simulink model "Furnace"  (R2020a)
settings: Solver=ode15s  StartTime=0  StopTime=27000  FixedStep=0.1  MaxStep=20  MinStep=1e-13  RelTol=1e-08  AbsTol=1e-09
undefined symbols (not defined in the file): agnostic_lqe_params, cont_reg, disturbance_type, F_aI_pid, F_aII_pid, input_type, k, lqe_params, LQR_params, LQRAgnostic_params, MPC_type, MPCDiscrete_function_parameters, MPCDiscreteAgnostic_function_parameters, MPCDiscreteDiffIntegralAgnostic_function_parameters, original_LQR_params, output_type, reg, single_butter_ss
libraries: simulink x35, cstblocks x10, mpclib x3
(part 2 of 8)

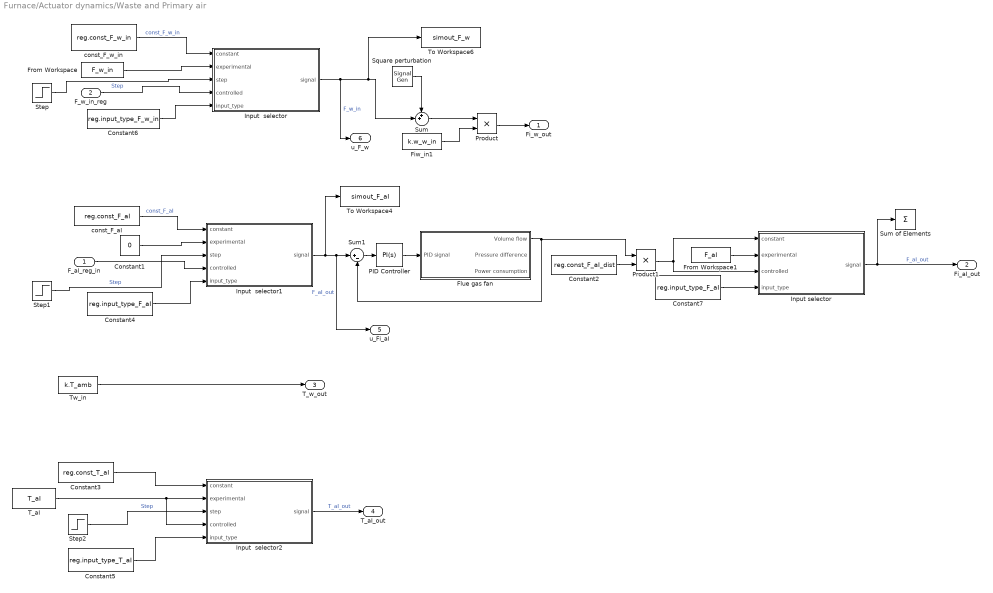
== system Furnace/Actuator dynamics/Waste and Primary air ==
  "F_aI_reg_in " : Inport
  F_w_in_reg : Inport  Port=2
  Constant1 : Constant  Value=0
  Constant2 : Constant  Value=reg.const_F_aI_dist
  Constant3 : Constant  Value=reg.const_T_aI
  Constant4 : Constant  Value=reg.input_type_F_aI
  Constant5 : Constant  Value=reg.input_type_T_aI
  Constant6 : Constant  Value=reg.input_type_F_w_in
  Constant7 : Constant  Value=reg.input_type_F_aI
  Fiw_in1 : Constant  Value=k.w_w_in
  Flue gas fan : Subsystem
  From Workspace : FromWorkspace  VariableName=F_w_in
  From Workspace1 : FromWorkspace  VariableName=F_aI
  Input  selector : MATLAB Function  TreatAsAtomicUnit=on
  Input  selector1 : MATLAB Function  TreatAsAtomicUnit=on
  Input  selector2 : MATLAB Function  TreatAsAtomicUnit=on
  Input selector : MATLAB Function  TreatAsAtomicUnit=on
  PID Controller : simulink/Continuous/PID Controller  Controller=PI  Form=Parallel  TimeDomain=Continuous-time  UseExternalTs=off  SampleTime=1  IntegratorMethod=Forward Euler  FilterMethod=Forward Euler  ControllerParametersSource=internal  P=reg.Kp_fan  I=reg.Ki_fan  D=0  UseFilter=on  N=100  TunerSelectOption=Transfer Function Based (PID Tuner App)  InitialConditionSource=internal  InitialConditionForIntegrator=reg.F_aI_fan_PID_int  InitialConditionForFilter=0  DifferentiatorICPrevScaledInput=0  ExternalReset=none  TrackingMode=off  Kt=1  LimitOutput=off  UpperSaturationLimit=inf  LowerSaturationLimit=-inf  LinearizeAsGain=on  AntiWindupMode=none  Kb=1  POutMin=[]  POutMax=[]  IOutMin=[]  IOutMax=[]  DOutMin=[]  DOutMax=[]  NOutMin=[]  NOutMax=[]  SumOutMin=[]  SumOutMax=[]  SaturationOutMin=[]  SaturationOutMax=[]  PParamMin=[]  PParamMax=[]  IParamMin=[]  IParamMax=[]  DParamMin=[]  DParamMax=[]  NParamMin=[]  NParamMax=[]  KbParamMin=[]  KbParamMax=[]  KtParamMin=[]  KtParamMax=[]  KbOutMin=[]  KbOutMax=[]  KtOutMin=[]  KtOutMax=[]  IntegratorOutMin=[]  IntegratorOutMax=[]  FilterOutMin=[]  FilterOutMax=[]  SumI1OutMin=[]  SumI1OutMax=[]  SumI2OutMin=[]  SumI2OutMax=[]  SumI3OutMin=[]  SumI3OutMax=[]  SumI4OutMin=[]  SumI4OutMax=[]  SumDOutMin=[]  SumDOutMax=[]  DifferentiatorOutMin=[]  DifferentiatorOutMax=[]  FilterDiffOutCoefMin=[]  FilterDiffOutCoefMax=[]  ReciprocalOutMin=[]  ReciprocalOutMax=[]  SumDenOutMin=[]  SumDenOutMax=[]  SumNumOutMin=[]  SumNumOutMax=[]  DivideOutMin=[]  DivideOutMax=[]  UdiffTsProdOutMin=[]  UdiffTsProdOutMax=[]  NTsProdOutMin=[]  NTsProdOutMax=[]  UintegralTsProdOutMin=[]  UintegralTsProdOutMax=[]  UngainTsProdOutMin=[]  UngainTsProdOutMax=[]  IntegratorContinuousStateAttributes=''  IntegratorStateMustResolveToSignalObject=off  IntegratorRTWStateStorageClass=Auto  FilterContinuousStateAttributes=''  FilterStateMustResolveToSignalObject=off  FilterRTWStateStorageClass=Auto  ParallelPVariant=InternalParameters  IdealPVariant=Disabled  IVariant=InternalParameters  DVariant=Disabled  IntegratorVariant=Continuous  SatVariant=Disabled  AWVariant=Passthrough  PCopyVariant=Disabled  TRVariant=Disabled  FdbkBlocksVariant=Forward  IdealPFdbkVariant=Disabled  SatFdbkVariant=Disabled  DerivativeFilterVariant=Disabled  NVariant=Disabled  NCopyVariant=Disabled_SignalSpec  FilterICVariant=Disabled  IntegratorICVariant=InternalICs  ExternalResetVariant=Disabled  TRSumVariant=Passthrough  SumFdbkVariant=Disabled  SumVariant=Sum_PI  TsampFilterVariant=InternalTs  TsampNgainVariant=Passthrough  TsampIntegralVariant=Passthrough
  Product : Product
  Product1 : Product
  Square perturbation : SignalGenerator  WaveForm=square  Amplitude=reg.F_w_pert_amp  Frequency=reg.F_w_pert_freq
  Step : Step  Time=reg.stepTime  Before=reg.const_F_w_in  After=reg.const_F_w_in_post_step  SampleTime=0
  Step1 : Step  Time=reg.stepTime  Before=reg.const_F_aI  After=reg.const_F_aI_post_step  SampleTime=0
  Step2 : Step  Time=reg.stepTime  Before=reg.const_T_aI  After=reg.const_T_aI_post_step  SampleTime=0
  Sum : Sum  Inputs=++|
  Sum of Elements : Sum  Inputs=+
  Sum1 : Sum  Inputs=|+-
  T_aI : FromWorkspace  VariableName=T_aI
  To Workspace4 : ToWorkspace  VariableName=simout_F_aI  SaveFormat=Timeseries  SampleTime=-1
  To Workspace6 : ToWorkspace  VariableName=simout_F_w  SaveFormat=Timeseries  SampleTime=-1
  Tw_in : Constant  Value=k.T_amb
  const_F_aI : Constant  Value=reg.const_F_aI
  const_F_w_in : Constant  Value=reg.const_F_w_in
  Fi_w_out : Outport  VectorParamsAs1DForOutWhenUnconnected=off
  Fi_aI_out : Outport  Port=2  VectorParamsAs1DForOutWhenUnconnected=off
  T_w_out : Outport  Port=3  VectorParamsAs1DForOutWhenUnconnected=off
  T_aI_out : Outport  Port=4  VectorParamsAs1DForOutWhenUnconnected=off
  u_Fi_aI : Outport  Port=5  VectorParamsAs1DForOutWhenUnconnected=off
  u_F_w : Outport  Port=6  VectorParamsAs1DForOutWhenUnconnected=off
  wires:
  Tw_in/1 -> T_w_out/1
  Fiw_in1/1 -> Product/2
  From Workspace/1 -> Input  selector/2(experimental)
  Product/1 -> Fi_w_out/1
  Input selector/1(signal) -> Fi_aI_out/1, Sum of Elements/1  "F_aI_out"
  From Workspace1/1 -> Input selector/2(experimental)
  Constant4/1 -> Input  selector1/5(input_type)
  Constant5/1 -> Input  selector2/5(input_type)
  T_aI/1 -> Input  selector2/4(controlled), Input  selector2/2(experimental)
  Constant3/1 -> Input  selector2/1(constant)
  Input  selector2/1(signal) -> T_aI_out/1  "T_aI_out"
  Constant6/1 -> Input  selector/5(input_type)
  F_w_in_reg/1 -> Input  selector/4(controlled)
  const_F_w_in/1 -> Input  selector/1(constant)  "const_F_w_in"
  Input  selector/1(signal) -> u_F_w/1, To Workspace6/1, Sum/2  "F_w_in"
  Sum/1 -> Product/1
  Square perturbation/1 -> Sum/1
  PID Controller/1 -> Flue gas fan/1(PID signal)
  Sum1/1 -> PID Controller/1
  const_F_aI/1 -> Input  selector1/1(constant)  "const_F_aI"
  "F_aI_reg_in "/1 -> Input  selector1/4(controlled)
  Constant1/1 -> Input  selector1/2(experimental)
  Constant2/1 -> Product1/2
  Product1/1 -> Input selector/1(constant), Input selector/3(controlled)
  Constant7/1 -> Input selector/4(input_type)
  Flue gas fan/1(Volume flow) -> Sum1/2, Product1/1
  Input  selector1/1(signal) -> To Workspace4/1, u_Fi_aI/1, Sum1/1  "F_aI_out"
  Step/1 -> Input  selector/3(step)  "Step"
  Step1/1 -> Input  selector1/3(step)  "Step"
  Step2/1 -> Input  selector2/3(step)  "Step"

== system Furnace/Controller/Butterworth_filter3 ==
  In : Inport
  Gain2 : Gain  Gain=single_butter_ss.B  Multiplication=Matrix(K*u)
  Gain3 : Gain  Gain=single_butter_ss.C  Multiplication=Matrix(K*u)
  Gain4 : Gain  Gain=single_butter_ss.A  Multiplication=Matrix(K*u)
  Integrator : Integrator
  Sum : Sum  Inputs=|++
  Filtered : Outport
  wires:
  Gain3/1 -> Filtered/1
  In/1 -> Gain2/1
  Gain2/1 -> Sum/1
  Integrator/1 -> Gain4/1, Gain3/1
  Gain4/1 -> Sum/2
  Sum/1 -> Integrator/1

== system Furnace/Controller/MPC_subsystem ==
  F_O2_in : Inport
  F_st_in : Inport  Port=2
  HHV_in : Inport  Port=3
  used_inputs : Inport  Port=4
  "\"Measured\" disturbances" : Inport  Port=5
  Constant1 : Constant  Value=lqe_params.u_star
  Constant11 : Constant  Value=lqe_params.y_star
  Constant2 : Constant  Value=lqe_params.u_star
  Constant3 : Constant  Value=lqe_params.v_star
  Demux1 : Demux
  LQG_controller : Subsystem
  MPC-ref : Constant  Value=[0;0]
  Mux2 : Mux  Inputs=3
  Revert to Summer ordering : Selector  InputPortWidth=4  IndexOptions=Index vector (dialog)  Indices=[1 3 4 2]  OutputSizes=1
  Scope{,1..4} (5 alike) : Scope
  Scope6 : Scope  Commented=on
  Selector : Selector  InputPortWidth=3  IndexOptions=Index vector (dialog)  Indices=[2 1 3]  OutputSizes=1
  Selector1 : Selector  InputPortWidth=3  IndexOptions=Index vector (dialog)  Indices=1:2  OutputSizes=1
  Selector5 : Selector  Commented=on  InputPortWidth=3  IndexOptions=Index vector (dialog)  Indices=1:2  OutputSizes=1
  Selector6 : Selector  InputPortWidth=5  IndexOptions=Index vector (dialog)  Indices=original_lqe_params.disturbance_measurement_indecies  OutputSizes=1
  Sine Wave : Sin  Commented=on  Amplitude=reg.include_noise * 1e-3  SampleTime=0
  Sum : Sum  Inputs=+-
  Sum1 : Sum  Inputs=|+-
  Sum2 : Sum  Inputs=|++
  Sum3 : Sum  Inputs=|+-
  Sum5 : Sum  Inputs=|+-
  Sum6 : Sum  Commented=on  Inputs=|-+
  Use internal ordering : Selector  InputPortWidth=4  IndexOptions=Index vector (dialog)  Indices=[1 4 2 3]  OutputSizes=1
  F_aII_MPC : Outport
  F_aI_MPC : Outport  Port=2
  v_grate_MPC : Outport  Port=3
  F_w_MPC : Outport  Port=4
  y_hat : Outport  Port=5
  wires:
  Demux1/1 -> F_aII_MPC/1
  Demux1/3 -> v_grate_MPC/1
  MPC-ref/1 -> LQG_controller/4(Controler_reference)
  Demux1/2 -> F_aI_MPC/1
  HHV_in/1 -> Mux2/3
  F_O2_in/1 -> Mux2/1
  F_st_in/1 -> Mux2/2
  Constant11/1 -> Sum1/2
  Demux1/4 -> F_w_MPC/1
  Sum2/1 -> Revert to Summer ordering/1
  Revert to Summer ordering/1 -> Demux1/1
  Selector/1 -> Sum1/1
  Selector1/1 -> Scope1/1  "MPC_y"
  Sum/1 -> Scope2/1
  Sum1/1 -> LQG_controller/1(noisy_y), Sum/2, Sum6/2, Selector1/1
  used_inputs/1 -> Use internal ordering/1
  Sum3/1 -> LQG_controller/3(u in)
  Constant2/1 -> Sum3/2
  Use internal ordering/1 -> Sum3/1
  Mux2/1 -> Selector/1
  Selector5/1 -> Scope6/1  "MPC_y"
  Sine Wave/1 -> Sum6/1
  Sum6/1 -> Selector5/1
  "\"Measured\" disturbances"/1 -> Selector6/1
  Constant3/1 -> Sum5/2
  Sum5/1 -> LQG_controller/2(v in), Scope4/1  "v in"
  Selector6/1 -> Sum5/1
  Constant1/1 -> Sum2/2
  LQG_controller/2(y_hat) -> y_hat/1, Scope3/1, Sum/1
  LQG_controller/1(u_mpc) -> Scope/1, Sum2/1

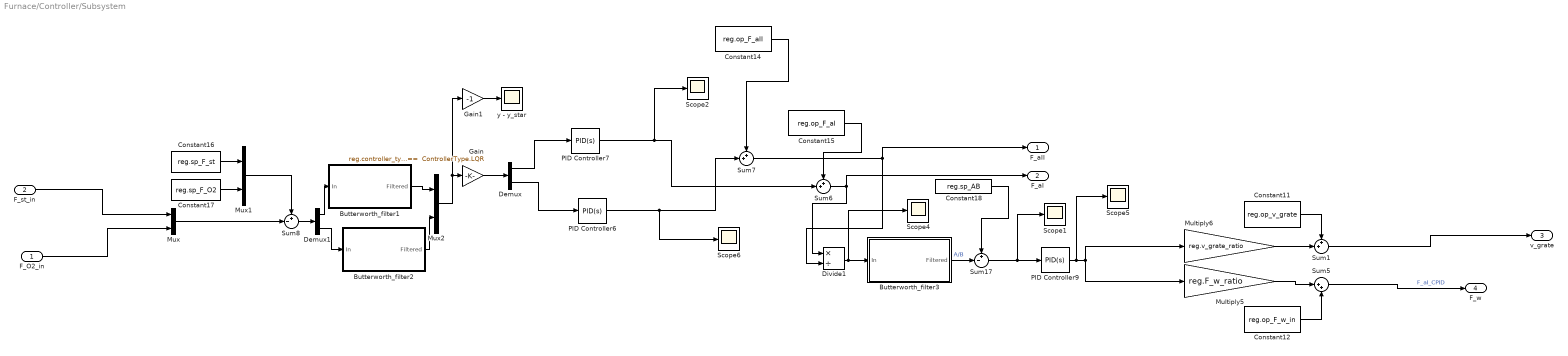
== system Furnace/Controller/Subsystem ==
  F_O2_in : Inport
  F_st_in : Inport  Port=2
  Butterworth_filter1 : Subsystem
  Butterworth_filter2 : Subsystem
  Butterworth_filter3 : Subsystem
  Constant11 : Constant  Value=reg.op_v_grate
  Constant12 : Constant  Value=reg.op_F_w_in
  Constant14 : Constant  Value=reg.op_F_aII
  Constant15 : Constant  Value=reg.op_F_aI
  Constant16 : Constant  Value=reg.sp_F_st
  Constant17 : Constant  Value=reg.sp_F_O2
  Constant18 : Constant  Value=reg.sp_AB
  Demux : Demux  Outputs=2
  Demux1 : Demux  Outputs=2
  Divide1 : Product  Inputs=*/
  Gain : Gain  Gain="reg.controller_type ==  ControllerType.LQR"
  Gain1 : Gain  Gain=-1
  Multiply5 : Gain  Gain=reg.F_w_ratio
  Multiply6 : Gain  Gain=reg.v_grate_ratio
  Mux : Mux  Inputs=2
  Mux1 : Mux  Inputs=2
  Mux2 : Mux  Inputs=2
  PID Controller6 : simulink/Continuous/PID Controller  Controller=PID  Form=Parallel  TimeDomain=Continuous-time  UseExternalTs=off  SampleTime=1  IntegratorMethod=Forward Euler  FilterMethod=Forward Euler  ControllerParametersSource=internal  P=F_aII_pid.Kp  I=F_aII_pid.Ki  D=F_aII_pid.Kd  UseFilter=on  N=100  TunerSelectOption=Transfer Function Based (PID Tuner App)  InitialConditionSource=internal  InitialConditionForIntegrator=0  InitialConditionForFilter=0  DifferentiatorICPrevScaledInput=0  ExternalReset=none  TrackingMode=off  Kt=1  LimitOutput=off  UpperSaturationLimit=inf  LowerSaturationLimit=1  LinearizeAsGain=on  AntiWindupMode=none  Kb=1  POutMin=[]  POutMax=[]  IOutMin=[]  IOutMax=[]  DOutMin=[]  DOutMax=[]  NOutMin=[]  NOutMax=[]  SumOutMin=[]  SumOutMax=[]  SaturationOutMin=[]  SaturationOutMax=[]  PParamMin=[]  PParamMax=[]  IParamMin=[]  IParamMax=[]  DParamMin=[]  DParamMax=[]  NParamMin=[]  NParamMax=[]  KbParamMin=[]  KbParamMax=[]  KtParamMin=[]  KtParamMax=[]  KbOutMin=[]  KbOutMax=[]  KtOutMin=[]  KtOutMax=[]  IntegratorOutMin=[]  IntegratorOutMax=[]  FilterOutMin=[]  FilterOutMax=[]  SumI1OutMin=[]  SumI1OutMax=[]  SumI2OutMin=[]  SumI2OutMax=[]  SumI3OutMin=[]  SumI3OutMax=[]  SumI4OutMin=[]  SumI4OutMax=[]  SumDOutMin=[]  SumDOutMax=[]  DifferentiatorOutMin=[]  DifferentiatorOutMax=[]  FilterDiffOutCoefMin=[]  FilterDiffOutCoefMax=[]  ReciprocalOutMin=[]  ReciprocalOutMax=[]  SumDenOutMin=[]  SumDenOutMax=[]  SumNumOutMin=[]  SumNumOutMax=[]  DivideOutMin=[]  DivideOutMax=[]  UdiffTsProdOutMin=[]  UdiffTsProdOutMax=[]  NTsProdOutMin=[]  NTsProdOutMax=[]  UintegralTsProdOutMin=[]  UintegralTsProdOutMax=[]  UngainTsProdOutMin=[]  UngainTsProdOutMax=[]  IntegratorContinuousStateAttributes='F_st'  IntegratorStateMustResolveToSignalObject=off  IntegratorRTWStateStorageClass=Auto  FilterContinuousStateAttributes=''  FilterStateMustResolveToSignalObject=off  FilterRTWStateStorageClass=Auto  ParallelPVariant=InternalParameters  IdealPVariant=Disabled  IVariant=InternalParameters  DVariant=InternalParameters  IntegratorVariant=Continuous  SatVariant=Disabled  AWVariant=Passthrough  PCopyVariant=Disabled  TRVariant=Disabled  FdbkBlocksVariant=Forward  IdealPFdbkVariant=Disabled  SatFdbkVariant=Disabled  DerivativeFilterVariant=ContFilter  NVariant=InternalParameters  NCopyVariant=Disabled  FilterICVariant=InternalICsFilter  IntegratorICVariant=InternalICs  ExternalResetVariant=Disabled  TRSumVariant=Passthrough  SumFdbkVariant=Disabled  SumVariant=Sum_PID  TsampFilterVariant=InternalTs  TsampNgainVariant=Passthrough  TsampIntegralVariant=Passthrough
  PID Controller7 : simulink/Continuous/PID Controller  Controller=PID  Form=Parallel  TimeDomain=Continuous-time  UseExternalTs=off  SampleTime=1  IntegratorMethod=Forward Euler  FilterMethod=Forward Euler  ControllerParametersSource=internal  P=F_aI_pid.Kp  I=F_aI_pid.Ki  D=F_aI_pid.Kd  UseFilter=on  N=100  TunerSelectOption=Transfer Function Based (PID Tuner App)  InitialConditionSource=internal  InitialConditionForIntegrator=0  InitialConditionForFilter=0  DifferentiatorICPrevScaledInput=0  ExternalReset=none  TrackingMode=off  Kt=1  LimitOutput=off  UpperSaturationLimit=inf  LowerSaturationLimit=1  LinearizeAsGain=on  AntiWindupMode=none  Kb=1  POutMin=[]  POutMax=[]  IOutMin=[]  IOutMax=[]  DOutMin=[]  DOutMax=[]  NOutMin=[]  NOutMax=[]  SumOutMin=[]  SumOutMax=[]  SaturationOutMin=[]  SaturationOutMax=[]  PParamMin=[]  PParamMax=[]  IParamMin=[]  IParamMax=[]  DParamMin=[]  DParamMax=[]  NParamMin=[]  NParamMax=[]  KbParamMin=[]  KbParamMax=[]  KtParamMin=[]  KtParamMax=[]  KbOutMin=[]  KbOutMax=[]  KtOutMin=[]  KtOutMax=[]  IntegratorOutMin=[]  IntegratorOutMax=[]  FilterOutMin=[]  FilterOutMax=[]  SumI1OutMin=[]  SumI1OutMax=[]  SumI2OutMin=[]  SumI2OutMax=[]  SumI3OutMin=[]  SumI3OutMax=[]  SumI4OutMin=[]  SumI4OutMax=[]  SumDOutMin=[]  SumDOutMax=[]  DifferentiatorOutMin=[]  DifferentiatorOutMax=[]  FilterDiffOutCoefMin=[]  FilterDiffOutCoefMax=[]  ReciprocalOutMin=[]  ReciprocalOutMax=[]  SumDenOutMin=[]  SumDenOutMax=[]  SumNumOutMin=[]  SumNumOutMax=[]  DivideOutMin=[]  DivideOutMax=[]  UdiffTsProdOutMin=[]  UdiffTsProdOutMax=[]  NTsProdOutMin=[]  NTsProdOutMax=[]  UintegralTsProdOutMin=[]  UintegralTsProdOutMax=[]  UngainTsProdOutMin=[]  UngainTsProdOutMax=[]  IntegratorContinuousStateAttributes='F_st'  IntegratorStateMustResolveToSignalObject=off  IntegratorRTWStateStorageClass=Auto  FilterContinuousStateAttributes=''  FilterStateMustResolveToSignalObject=off  FilterRTWStateStorageClass=Auto  ParallelPVariant=InternalParameters  IdealPVariant=Disabled  IVariant=InternalParameters  DVariant=InternalParameters  IntegratorVariant=Continuous  SatVariant=Disabled  AWVariant=Passthrough  PCopyVariant=Disabled  TRVariant=Disabled  FdbkBlocksVariant=Forward  IdealPFdbkVariant=Disabled  SatFdbkVariant=Disabled  DerivativeFilterVariant=ContFilter  NVariant=InternalParameters  NCopyVariant=Disabled  FilterICVariant=InternalICsFilter  IntegratorICVariant=InternalICs  ExternalResetVariant=Disabled  TRSumVariant=Passthrough  SumFdbkVariant=Disabled  SumVariant=Sum_PID  TsampFilterVariant=InternalTs  TsampNgainVariant=Passthrough  TsampIntegralVariant=Passthrough
  PID Controller9 : simulink/Continuous/PID Controller  Controller=PID  Form=Parallel  TimeDomain=Continuous-time  UseExternalTs=off  SampleTime=1  IntegratorMethod=Forward Euler  FilterMethod=Forward Euler  ControllerParametersSource=internal  P=F_aII_pid.Kp  I=F_aII_pid.Ki  D=F_aII_pid.Kd  UseFilter=on  N=100  TunerSelectOption=Transfer Function Based (PID Tuner App)  InitialConditionSource=internal  InitialConditionForIntegrator=0  InitialConditionForFilter=0  DifferentiatorICPrevScaledInput=0  ExternalReset=none  TrackingMode=off  Kt=1  LimitOutput=off  UpperSaturationLimit=inf  LowerSaturationLimit=1  LinearizeAsGain=on  AntiWindupMode=none  Kb=1  POutMin=[]  POutMax=[]  IOutMin=[]  IOutMax=[]  DOutMin=[]  DOutMax=[]  NOutMin=[]  NOutMax=[]  SumOutMin=[]  SumOutMax=[]  SaturationOutMin=[]  SaturationOutMax=[]  PParamMin=[]  PParamMax=[]  IParamMin=[]  IParamMax=[]  DParamMin=[]  DParamMax=[]  NParamMin=[]  NParamMax=[]  KbParamMin=[]  KbParamMax=[]  KtParamMin=[]  KtParamMax=[]  KbOutMin=[]  KbOutMax=[]  KtOutMin=[]  KtOutMax=[]  IntegratorOutMin=[]  IntegratorOutMax=[]  FilterOutMin=[]  FilterOutMax=[]  SumI1OutMin=[]  SumI1OutMax=[]  SumI2OutMin=[]  SumI2OutMax=[]  SumI3OutMin=[]  SumI3OutMax=[]  SumI4OutMin=[]  SumI4OutMax=[]  SumDOutMin=[]  SumDOutMax=[]  DifferentiatorOutMin=[]  DifferentiatorOutMax=[]  FilterDiffOutCoefMin=[]  FilterDiffOutCoefMax=[]  ReciprocalOutMin=[]  ReciprocalOutMax=[]  SumDenOutMin=[]  SumDenOutMax=[]  SumNumOutMin=[]  SumNumOutMax=[]  DivideOutMin=[]  DivideOutMax=[]  UdiffTsProdOutMin=[]  UdiffTsProdOutMax=[]  NTsProdOutMin=[]  NTsProdOutMax=[]  UintegralTsProdOutMin=[]  UintegralTsProdOutMax=[]  UngainTsProdOutMin=[]  UngainTsProdOutMax=[]  IntegratorContinuousStateAttributes='F_st'  IntegratorStateMustResolveToSignalObject=off  IntegratorRTWStateStorageClass=Auto  FilterContinuousStateAttributes=''  FilterStateMustResolveToSignalObject=off  FilterRTWStateStorageClass=Auto  ParallelPVariant=InternalParameters  IdealPVariant=Disabled  IVariant=InternalParameters  DVariant=InternalParameters  IntegratorVariant=Continuous  SatVariant=Disabled  AWVariant=Passthrough  PCopyVariant=Disabled  TRVariant=Disabled  FdbkBlocksVariant=Forward  IdealPFdbkVariant=Disabled  SatFdbkVariant=Disabled  DerivativeFilterVariant=ContFilter  NVariant=InternalParameters  NCopyVariant=Disabled  FilterICVariant=InternalICsFilter  IntegratorICVariant=InternalICs  ExternalResetVariant=Disabled  TRSumVariant=Passthrough  SumFdbkVariant=Disabled  SumVariant=Sum_PID  TsampFilterVariant=InternalTs  TsampNgainVariant=Passthrough  TsampIntegralVariant=Passthrough
  Scope{1..2,4..6} (5 alike) : Scope
  Sum1 : Sum  Inputs=++|
  Sum17 : Sum  Inputs=+-|
  Sum5 : Sum  Inputs=|++
  Sum6 : Sum  Inputs=++|
  Sum7 : Sum  Inputs=++|
  Sum8 : Sum  Inputs=+-|
  y - y_star : Scope
  F_aII : Outport
  F_aI : Outport  Port=2
  v_grate : Outport  Port=3
  F_w : Outport  Port=4
  wires:
  Gain/1 -> Demux/1
  Constant14/1 -> Sum7/1
  Demux1/2 -> Butterworth_filter2/1(In)
  PID Controller6/1 -> Scope6/1, Sum7/2
  PID Controller7/1 -> Scope2/1, Sum6/2
  Sum17/1 -> Scope1/1, PID Controller9/1
  Constant11/1 -> Sum1/1
  Constant18/1 -> Sum17/1
  Demux/2 -> PID Controller6/1
  Mux/1 -> Sum8/2
  Constant16/1 -> Mux1/1
  Multiply6/1 -> Sum1/2
  Constant15/1 -> Sum6/1
  Sum8/1 -> Demux1/1
  Sum6/1 -> F_aI/1, Divide1/1
  Constant17/1 -> Mux1/2
  Demux/1 -> PID Controller7/1
  Multiply5/1 -> Sum5/1
  Butterworth_filter3/1(Filtered) -> Sum17/2  "A/B"
  F_O2_in/1 -> Mux/2
  Sum1/1 -> v_grate/1
  Mux1/1 -> Sum8/1
  F_st_in/1 -> Mux/1
  PID Controller9/1 -> Scope5/1, Multiply5/1, Multiply6/1
  Sum7/1 -> F_aII/1, Divide1/2
  Sum5/1 -> F_w/1  "F_aI_CPID"
  Mux2/1 -> Gain1/1, Gain/1
  Butterworth_filter1/1(Filtered) -> Mux2/1
  Divide1/1 -> Butterworth_filter3/1(In), Scope4/1
  Demux1/1 -> Butterworth_filter1/1(In)
  Constant12/1 -> Sum5/2
  Butterworth_filter2/1(Filtered) -> Mux2/2
  Gain1/1 -> y - y_star/1

== system Furnace/Deprecated, slow loop/Actuator dynamics ==
  F_aII_reg_in : Inport
  F_w_in_reg : Inport  Port=2
  "F_aI_reg_in " : Inport  Port=3
  v_grate_reg_in : Inport  Port=4
  uncontrolled_variables : Inport  Port=5
  Bus Selector : BusSelector  OutputSignals=Q_grate,Tw,T_aI,T_aII
  Grate speed : Subsystem
  Secondary air : Subsystem
      mask Display: image('airflow.jpeg');
  Waste and Primary air : Subsystem
      mask Display: image('waste_in.jpg');
  v_grate : Outport
  Q_grate_out : Outport  Port=2
  Fi_w : Outport  Port=3
  Fi_aI : Outport  Port=4
  T_w : Outport  Port=5
  T_aI : Outport  Port=6
  F_aII_out : Outport  Port=7
  T_aII_out : Outport  Port=8
  wires:
  Grate speed/1(v_grate_out) -> v_grate/1  "v_grate"
  F_w_in_reg/1 -> Waste and Primary air/2(F_w_in_reg)
  Secondary air/1(F_aII_out) -> F_aII_out/1
  v_grate_reg_in/1 -> Grate speed/1(v_grate_reg_in)
  Waste and Primary air/1(Fi_w_out) -> Fi_w/1  "Fi_w"
  "F_aI_reg_in "/1 -> Waste and Primary air/1("F_aI_reg_in ")
  Waste and Primary air/2(Fi_aI_out) -> Fi_aI/1  "Fi_aI"
  F_aII_reg_in/1 -> Secondary air/1(F_aII_reg_in)
  uncontrolled_variables/1 -> Bus Selector/1
  Bus Selector/1 -> Q_grate_out/1  "<Q_grate>"
  Bus Selector/2 -> T_w/1  "<Tw>"
  Bus Selector/3 -> T_aI/1  "<T_aI>"
  Bus Selector/4 -> T_aII_out/1  "<T_aII>"

== system Furnace/Deprecated, slow loop/Constant disturbances ==
  Constant2 : Constant  Value=reg.const_T_aII
  Constant3 : Constant  Value=reg.const_T_aI
  Tw_in : Constant  Value=k.T_amb
  const_Q_grate : Constant  Value=reg.const_Q_grate
  Q_grate : Outport
  T_w : Outport  Port=2
  T_aI : Outport  Port=3
  T_aII : Outport  Port=4
  wires:
  Constant2/1 -> T_aII/1  "T_aII"
  const_Q_grate/1 -> Q_grate/1  "Q_grate"
  Tw_in/1 -> T_w/1  "Tw"
  Constant3/1 -> T_aI/1  "T_aI"

== system Furnace/Deprecated, slow loop/Constant inputs ==
  F_aII distribution : Gain  Gain=reg.const_F_aI_dist
  const_F_aI : Constant  Value=reg.const_F_aI
  const_F_aII : Constant  Value=reg.const_F_aII
  const_F_w_in : Constant  Value=reg.const_F_w_in
  const_v_grate : Constant  Value=reg.const_v_grate
  F_aII : Outport
  Fw : Outport  Port=2
  F_aI : Outport  Port=3
  v_grate : Outport  Port=4
  wires:
  const_v_grate/1 -> v_grate/1  "v_grate"
  const_F_aII/1 -> F_aII/1  "F_aII"
  const_F_aI/1 -> F_aII distribution/1  "F_aI"
  const_F_w_in/1 -> Fw/1  "F_w"
  F_aII distribution/1 -> F_aI/1  "F_aI"

== system Furnace/Deprecated, slow loop/Contineous Summer student feedback (Not finished) ==
  Fi_fg_in : Inport
  F_st_in : Inport  Port=2
  HHV_in : Inport  Port=3
  Controller : Subsystem
  Grate speed : Subsystem
  Secondary air : Subsystem
      mask Display: image('airflow.jpeg');
  Terminator{1..4} (4 alike) : Terminator
  Waste and Primary air : Subsystem
      mask Display: image('waste_in.jpg');
  F_aII_out : Outport
  Fi_w : Outport  Port=2
  Fi_aI : Outport  Port=3
  v_grate : Outport  Port=4
  wires:
  Controller/4(Fi_w_out) -> Waste and Primary air/2(F_w_in_reg)
  Controller/3(v_grate_out) -> Grate speed/1(v_grate_reg_in)
  Secondary air/1(F_aII_out) -> F_aII_out/1
  F_st_in/1 -> Controller/2(F_st_in)
  Fi_fg_in/1 -> Controller/1(Fi_fg_in)
  HHV_in/1 -> Controller/3(HHV_in)
  Grate speed/1(v_grate_out) -> v_grate/1  "v_grate"
  Controller/2(Fi_aI_out) -> Waste and Primary air/1("F_aI_reg_in ")
  Waste and Primary air/2(Fi_aI_out) -> Fi_aI/1  "Fi_aI"
  Controller/1(F_aII_out) -> Secondary air/1(F_aII_reg_in)
  Waste and Primary air/1(Fi_w_out) -> Fi_w/1  "Fi_w"
  Waste and Primary air/3(Fi_aI_out1) -> Terminator2/1
  Waste and Primary air/4(Fi_aI_out2) -> Terminator1/1
  Secondary air/2(F_aII_out1) -> Terminator3/1
  Grate speed/2(Q_grate_out) -> Terminator4/1

== system Furnace/Deprecated, slow loop/Controller ==
  F_st_in : Inport
  Fi_fg_in : Inport  Port=2
  HHV_in : Inport  Port=3
  Summer Controller (Cleaned) : Subsystem
  "Summer Controller (Old) " : Subsystem  Commented=on
  F_aII_out : Outport
  Fi_w_out : Outport  Port=2
  Full_Fi_aI_out : Outport  Port=3
  v_grate_out : Outport  Port=4
  wires:
  F_st_in/1 -> Summer Controller (Cleaned)/1(F_st_in)
  Fi_fg_in/1 -> Summer Controller (Cleaned)/2(Fi_O2_in)
  HHV_in/1 -> Summer Controller (Cleaned)/3(HHV_in)
  Summer Controller (Cleaned)/1(F_aII_out) -> F_aII_out/1
  Summer Controller (Cleaned)/3(Fi_aI_out) -> Full_Fi_aI_out/1
  Summer Controller (Cleaned)/2(Fi_w_out) -> Fi_w_out/1
  Summer Controller (Cleaned)/4(v_grate_out) -> v_grate_out/1

== system Furnace/Deprecated, slow loop/Experimental disturbances ==
  Constant  T_amb : Constant  Value=k.T_amb
  From Workspace2 : FromWorkspace  VariableName=Q_grate
  T_aII : FromWorkspace  VariableName=T_aII
  T_aI_w : FromWorkspace  VariableName=T_aI
  Q_grate1 : Outport
  T_w : Outport  Port=2
  T_aI1 : Outport  Port=3
  T_aII2 : Outport  Port=4
  wires:
  T_aII/1 -> T_aII2/1  "T_aII"
  From Workspace2/1 -> Q_grate1/1  "Q_grate"
  T_aI_w/1 -> T_aI1/1  "T_aI"
  Constant  T_amb/1 -> T_w/1  "Tw"

== system Furnace/Deprecated, slow loop/Experimental inputs ==
  Constant2 : Constant  Value=reg.const_F_aI_dist
  From Workspace : FromWorkspace  VariableName=F_w_in
  From Workspace1 : FromWorkspace  VariableName=F_aII
  From Workspace3 : FromWorkspace  VariableName=F_aI
  v_grate1 : Constant  Value=k.v_grate
  F_aII : Outport
  Fw : Outport  Port=2
  F_aI : Outport  Port=3
  v_grate : Outport  Port=4
  wires:
  From Workspace1/1 -> F_aII/1  "F_aII"
  From Workspace3/1 -> F_aI/1  "F_aI"
  v_grate1/1 -> v_grate/1  "v_grate"
  From Workspace/1 -> Fw/1  "F_w"

== system Furnace/Deprecated, slow loop/Furnace ==
  v_grate_in : Inport
  Q_grate_in : Inport  Port=2
  Fi_w_in : Inport  Port=3
  Fi_aI_in : Inport  Port=4
  T_w_in : Inport  Port=5
  T_aI_in : Inport  Port=6
  F_aII_in : Inport  Port=7
  T_aII_in : Inport  Port=8
  Ashes : Subsystem
      mask Display: image('ash.jpg');
  "Auxiliary \"burners\"" : Subsystem
      mask Display: image('burnerim.jpg');
  Boiler : Subsystem
      mask Display: image('Boiler.jpg');
  Bus Selector : BusSelector  OutputSignals=F_w_ash
  Calorific Value : Subsystem
  Cold water from district heating : Subsystem
      mask Display: image('fromdh.jpg');
  Condenser : Subsystem
      mask Display: image('Condenser.jpg');
  Flue-gas fan : Subsystem  Commented=on
      mask Display: image('Fan.jpg');
  Flue-gas stack : Subsystem  Commented=on
      mask Display: image('Stack.jpg');
  Free board : Subsystem
      mask Display: image('fbim.jpg');
  Gas cleaning systems : Subsystem  Commented=on
      mask Display: image('Cleaning.jpg');
  Grate : Subsystem
      settings: MinAlgLoopOccurrences=on
      mask Display: image('grateim.jpg');
  Hot water to district heating : Subsystem
      mask Display: image('todh.jpg');
  Scope : Scope
  Scope1 : Scope
  Scope2 : Scope
  Turbine : Subsystem
      mask Display: image('Turbine.jpg');
  F_st_out : Outport  VectorParamsAs1DForOutWhenUnconnected=off
  F_fg_out : Outport  Port=2  VectorParamsAs1DForOutWhenUnconnected=off
  HHV_out : Outport  Port=3  VectorParamsAs1DForOutWhenUnconnected=off
  wires:
  Boiler/3(p_drum) -> Turbine/3(p_drum)
  Free board/1(T_fg_out) -> Calorific Value/1(T_fg), Scope/1, Boiler/2(T_fg), Grate/1(T_rad), "Auxiliary \"burners\""/1(In1)  "T_rad"
  Turbine/1(F_turb) -> Condenser/2(F_turb)
  Grate/1(Fi_fg_from_grate) -> Ashes/1(In1), Free board/1(Fi_in)
  Q_grate_in/1 -> Grate/4(Q_grate)
  Condenser/1(T_district) -> Hot water to district heating/1(In1)
  Cold water from district heating/1(Out1) -> Condenser/1(F_district)
  Grate/2(T_w_grate) -> Ashes/2(In2), Free board/2(T_in)
  "Auxiliary \"burners\""/1(Out1) -> Scope1/1, Grate/2(Q_burners)  "Q_burners"
  Grate/4(Q_rad_fg) -> Free board/3(Q_rad)
  Free board/2(Fi_fg_to_boiler) -> F_fg_out/1, Calorific Value/2(Fi_fg), Boiler/3(F_fg)
  Flue-gas fan/1(Out1) -> Flue-gas stack/1(T_fg)
  Boiler/4(T_fg_out) -> Gas cleaning systems/1(T_fg)
  Boiler/2(F_SH) -> F_st_out/1, Turbine/2(F_SH)  "F_steam"
  Flue-gas fan/2(Out2) -> Flue-gas stack/2(Fi_fg)
  Grate/5(OutBus) -> Bus Selector/1, Ashes/3(InBus)
  Condenser/2(T_w_out) -> Boiler/1(T_fromHE)
  Gas cleaning systems/2(Fi_fg_clean) -> Flue-gas fan/2(Fi_fg)
  Boiler/1(T_SH) -> Turbine/1(T_SH)
  Free board/3(F_flyash_tot) -> Boiler/4(F_flyash)
  Grate/3(F_flyash) -> Free board/4(F_flyash_cell)
  Gas cleaning systems/1(T_fg_clean) -> Flue-gas fan/1(T_fg)
  v_grate_in/1 -> Grate/3(v_grate_in)
  Boiler/5(Fi_fg_out) -> Gas cleaning systems/2(F_fg)
  Condenser/3(F_cond) -> Boiler/5(F_ECO)
  Boiler/6(F_flyash_out) -> Gas cleaning systems/3(F_flyash)
  Cold water from district heating/2(Out2) -> Condenser/3(T_return)
  Calorific Value/1(HHV) -> HHV_out/1  "HHV"
  Fi_w_in/1 -> Grate/5(Fi_w_in)
  Fi_aI_in/1 -> Grate/6(F_aI_in)
  T_w_in/1 -> Grate/7(T_w_in)
  T_aI_in/1 -> Grate/8(T_aI_in)
  F_aII_in/1 -> Free board/5(F_aII_in)
  T_aII_in/1 -> Free board/6(T_aII_in)
  Bus Selector/1 -> Scope2/1  "<F_w_ash>"

== system Furnace/Plant2/Ashes ==
  In1 : Inport
  In2 : Inport  Port=2
  In Bus Element : Inport  Port=3  PortName=InBus  Element=M_w_grate
  In Bus Element1 : Inport  Port=3  PortName=InBus  Element=M_char
  In Bus Element2 : Inport  Port=3  PortName=InBus  Element=F_w_ash
  In Bus Element3 : Inport  Port=3  PortName=InBus  Element=F_char_ash
  Flow of char ash : Display
  Flow of waste ash : Display
  Mass of char in grate : Display
  Scope1 : Scope
  Sum of Elements : Sum  Inputs=+  CollapseMode=Specified dimension
  Temperatures in grate : Display
  Waste in grate (mass) : Display
  wires:
  In Bus Element2/1 -> Flow of waste ash/1
  In Bus Element/1 -> Waste in grate (mass)/1
  In Bus Element1/1 -> Mass of char in grate/1
  In Bus Element3/1 -> Flow of char ash/1
  In1/1 -> Sum of Elements/1
  In2/1 -> Temperatures in grate/1
  Sum of Elements/1 -> Scope1/1

== system Furnace/Plant2/Auxiliary "burners" ==
  In1 : Inport
  Constant : Constant  Value=0
  Constant1 : Constant  Value=850+k.T_amb
  Minus : Sum  Inputs=+-
  "Q " : Constant  Value=3.5e6
  Switch : Switch  Criteria=u2 > Threshold
  Out1 : Outport  VectorParamsAs1DForOutWhenUnconnected=off
  wires:
  Switch/1 -> Out1/1
  Constant/1 -> Switch/3
  "Q "/1 -> Switch/1
  Minus/1 -> Switch/2
  Constant1/1 -> Minus/1
  In1/1 -> Minus/2

== system Furnace/Plant2/Boiler ==
  T_fromHE : Inport
  T_fg : Inport  Port=2
  F_fg : Inport  Port=3
  F_flyash : Inport  Port=4
  F_ECO : Inport  Port=5
  Constant : Constant  Value=0
  Constant1 : Constant  Value=k.p_drum
  Constant2 : Constant  Value=k.p_drum
  Drum : Subsystem
      mask Display: image('Drum.jpg');
  Economizer : Subsystem
  Evaporator : Subsystem
  Gain : Gain  Gain=1e-5
  Goto : Goto  Commented=on  GotoTag=T_drum  TagVisibility=global
  MATLAB Function : MATLAB Function  TreatAsAtomicUnit=on
  PID Controller : simulink/Continuous/PID Controller  Controller=PID  Form=Parallel  TimeDomain=Continuous-time  UseExternalTs=off  SampleTime=-1  IntegratorMethod=Forward Euler  FilterMethod=Forward Euler  ControllerParametersSource=internal  P=10  I=0  D=0  UseFilter=on  N=100  TunerSelectOption=Transfer Function Based (PID Tuner App)  InitialConditionSource=internal  InitialConditionForIntegrator=0  InitialConditionForFilter=0  DifferentiatorICPrevScaledInput=0  ExternalReset=none  TrackingMode=off  Kt=1  LimitOutput=on  UpperSaturationLimit=50  LowerSaturationLimit=0  LinearizeAsGain=on  AntiWindupMode=none  Kb=1  POutMin=[]  POutMax=[]  IOutMin=[]  IOutMax=[]  DOutMin=[]  DOutMax=[]  NOutMin=[]  NOutMax=[]  SumOutMin=[]  SumOutMax=[]  SaturationOutMin=[]  SaturationOutMax=[]  PParamMin=[]  PParamMax=[]  IParamMin=[]  IParamMax=[]  DParamMin=[]  DParamMax=[]  NParamMin=[]  NParamMax=[]  KbParamMin=[]  KbParamMax=[]  KtParamMin=[]  KtParamMax=[]  KbOutMin=[]  KbOutMax=[]  KtOutMin=[]  KtOutMax=[]  IntegratorOutMin=[]  IntegratorOutMax=[]  FilterOutMin=[]  FilterOutMax=[]  SumI1OutMin=[]  SumI1OutMax=[]  SumI2OutMin=[]  SumI2OutMax=[]  SumI3OutMin=[]  SumI3OutMax=[]  SumI4OutMin=[]  SumI4OutMax=[]  SumDOutMin=[]  SumDOutMax=[]  DifferentiatorOutMin=[]  DifferentiatorOutMax=[]  FilterDiffOutCoefMin=[]  FilterDiffOutCoefMax=[]  ReciprocalOutMin=[]  ReciprocalOutMax=[]  SumDenOutMin=[]  SumDenOutMax=[]  SumNumOutMin=[]  SumNumOutMax=[]  DivideOutMin=[]  DivideOutMax=[]  UdiffTsProdOutMin=[]  UdiffTsProdOutMax=[]  NTsProdOutMin=[]  NTsProdOutMax=[]  UintegralTsProdOutMin=[]  UintegralTsProdOutMax=[]  UngainTsProdOutMin=[]  UngainTsProdOutMax=[]  IntegratorContinuousStateAttributes=''  IntegratorStateMustResolveToSignalObject=off  IntegratorRTWStateStorageClass=Auto  FilterContinuousStateAttributes=''  FilterStateMustResolveToSignalObject=off  FilterRTWStateStorageClass=Auto  ParallelPVariant=InternalParameters  IdealPVariant=Disabled  IVariant=InternalParameters  DVariant=InternalParameters  IntegratorVariant=Continuous  SatVariant=Enabled  AWVariant=Passthrough  PCopyVariant=Disabled  TRVariant=Disabled  FdbkBlocksVariant=Forward  IdealPFdbkVariant=Disabled  SatFdbkVariant=Disabled  DerivativeFilterVariant=ContFilter  NVariant=InternalParameters  NCopyVariant=Disabled  FilterICVariant=InternalICsFilter  IntegratorICVariant=InternalICs  ExternalResetVariant=Disabled  TRSumVariant=Passthrough  SumFdbkVariant=Disabled  SumVariant=Sum_PID  TsampFilterVariant=InternalTs  TsampNgainVariant=Passthrough  TsampIntegralVariant=Passthrough
  PID null saturator : Switch
  Scope : Scope
  Scope1 : Scope
  Scope2 : Scope
  Sum1 : Sum  Inputs=+-|
  Super heater : Subsystem
  x_vap : Scope
  T_SH : Outport  VectorParamsAs1DForOutWhenUnconnected=off
  F_SH : Outport  Port=2  PortDimensions=1  VectorParamsAs1DForOutWhenUnconnected=off
  p_drum : Outport  Port=3  VectorParamsAs1DForOutWhenUnconnected=off
  T_fg_out : Outport  Port=4  VectorParamsAs1DForOutWhenUnconnected=off
  Fi_fg_out : Outport  Port=5  VectorParamsAs1DForOutWhenUnconnected=off
  F_flyash_out : Outport  Port=6  VectorParamsAs1DForOutWhenUnconnected=off
  wires:
  Evaporator/3(Fi_fg_out) -> Super heater/4(Fi_fg)
  Super heater/4(Fi_fg_out) -> Economizer/3(Fi_fg)
  Super heater/3(T_fg_out) -> Economizer/2(T_fg)
  Evaporator/2(T_fg_out) -> Super heater/3(T_fg)
  Economizer/3(Fi_fg_out) -> Fi_fg_out/1
  F_fg/1 -> Evaporator/3(Fi_fg)
  T_fg/1 -> Evaporator/2(T_fg)
  Super heater/2(T_steam) -> T_SH/1
  Economizer/2(T_fg_out) -> T_fg_out/1
  Drum/3(p_drum) -> MATLAB Function/1(p_drum), Sum1/1, p_drum/1
  T_fromHE/1 -> Economizer/1(T_fromHE)
  Super heater/5(F_SH) -> F_SH/1
  Drum/2(x_vap) -> x_vap/1
  PID Controller/1 -> Drum/3(F_vap), Scope/1, Super heater/1(F_steam)
  Constant1/1 -> Sum1/2
  Constant/1 -> PID null saturator/3
  Sum1/1 -> Gain/1
  [Q_cleaning] -> Drum/5(Q_cleaning)
  F_flyash/1 -> F_flyash_out/1
  Super heater/1(Q_SH) -> Scope1/1
  Economizer/1(Q_ECO) -> Scope2/1
  Economizer/4(F_ECO) -> Drum/1(F_ECO)
  Evaporator/1(Q_EVA) -> Drum/2(Q_EVA)
  Economizer/5(T_ECO2) -> Drum/4(T_ECO)
  F_ECO/1 -> Economizer/4(F_w)
  PID null saturator/1 -> PID Controller/1
  Gain/1 -> PID null saturator/1
  Drum/1(T_drum) -> Goto/1, Super heater/2(T_drum), Evaporator/1(T_drum)
  MATLAB Function/1(switch_on) -> PID null saturator/2
  Constant2/1 -> MATLAB Function/2(k_p_drum)

== system Furnace/Plant2/Calorific Value ==
  T_fg : Inport
  Fi_fg : Inport  Port=2
  MATLAB Function : MATLAB Function  TreatAsAtomicUnit=on
  T_amb : Constant  Value=k.T_amb
  cp_fg : Constant  Value=k.cp_fg
  HHV : Outport  VectorParamsAs1DForOutWhenUnconnected=off
  wires:
  cp_fg/1 -> MATLAB Function/3(cp_fg)
  Fi_fg/1 -> MATLAB Function/1(Fi_fg)
  T_amb/1 -> MATLAB Function/4(T_amb)
  MATLAB Function/1(HHV) -> HHV/1
  T_fg/1 -> MATLAB Function/2(T_fg)
  [F_aI] -> MATLAB Function/5(F_aI)
  [T_aI] -> MATLAB Function/6(T_aI)
  [F_aII] -> MATLAB Function/7(F_aII)
  [T_aII] -> MATLAB Function/8(T_aII)

== system Furnace/Plant2/Cold water from district heating ==
  Constant : Constant  Value=reg.const_F_from_DH
  Constant2 : Constant  Value=reg.const_T_from_DH
  From Workspace1 : FromWorkspace  VariableName=F_from_DH
  From Workspace2 : FromWorkspace  VariableName=T_from_DH
  Selector : Selector  InputPortWidth=2  IndexOptions=Index vector (dialog)  Indices=reg.input_type_F_from_DH  OutputSizes=1
  Selector1 : Selector  InputPortWidth=2  IndexOptions=Index vector (dialog)  Indices=reg.input_type_T_from_DH  OutputSizes=1
  Vector Concatenate : Concatenate
  Vector Concatenate1 : Concatenate
  Out1 : Outport  VectorParamsAs1DForOutWhenUnconnected=off
  Out2 : Outport  Port=2  VectorParamsAs1DForOutWhenUnconnected=off
  wires:
  From Workspace1/1 -> Vector Concatenate/2
  Constant/1 -> Vector Concatenate/1
  Constant2/1 -> Vector Concatenate1/1
  From Workspace2/1 -> Vector Concatenate1/2
  Vector Concatenate/1 -> Selector/1
  Selector/1 -> Out1/1  "F_from_DH"
  Vector Concatenate1/1 -> Selector1/1
  Selector1/1 -> Out2/1  "T_from_DH"

== system Furnace/Plant2/Condenser ==
  F_district : Inport
  F_turb : Inport  Port=2
  T_return : Inport  Port=3
  Constant : Constant  Value=k.cp_water
  Constant1 : Constant  Value=k.epsilon_HE
  Constant2 : Constant  Value=k.eff_HE
  District heating heat exchanger : MATLAB Function  TreatAsAtomicUnit=on
  Scope : Scope
  Transport Delay1 : TransportDelay  DelayTime=2
  Transport Delay2 : TransportDelay  DelayTime=2  InitialOutput=k.T_amb  BufferSize=2048
  Transport Delay3 : TransportDelay  DelayTime=2  InitialOutput=k.T_amb
  Transport Delay4 : TransportDelay  DelayTime=2  InitialOutput=k.T_amb
  p_HP : Constant  Value=k.p_HP
  T_district : Outport  VectorParamsAs1DForOutWhenUnconnected=off
  T_w_out : Outport  Port=2  VectorParamsAs1DForOutWhenUnconnected=off
  F_cond : Outport  Port=3  VectorParamsAs1DForOutWhenUnconnected=off
  wires:
  F_district/1 -> District heating heat exchanger/1(F_DH)
  p_HP/1 -> District heating heat exchanger/2(p_HP)
  T_return/1 -> District heating heat exchanger/4(T_return)
  Constant/1 -> District heating heat exchanger/5(cp_water)
  Constant1/1 -> District heating heat exchanger/6(epsilon_HE)
  District heating heat exchanger/1(Q_HE) -> Transport Delay1/1
  District heating heat exchanger/3(T_district) -> Transport Delay3/1
  District heating heat exchanger/2(Tw_ECO) -> Transport Delay2/1
  F_turb/1 -> Transport Delay4/1, District heating heat exchanger/3(F_turb)
  Transport Delay1/1 -> Scope/1
  Transport Delay2/1 -> T_w_out/1
  Transport Delay3/1 -> T_district/1
  Constant2/1 -> District heating heat exchanger/7(eff_HE)
  Transport Delay4/1 -> F_cond/1

== system Furnace/Plant2/Flue-gas fan ==
  T_fg : Inport
  Fi_fg : Inport  Port=2
  Fan : MATLAB Function  TreatAsAtomicUnit=on
  Sum of Elements : Sum  Inputs=+
  Out1 : Outport  VectorParamsAs1DForOutWhenUnconnected=off
  Out2 : Outport  Port=2  VectorParamsAs1DForOutWhenUnconnected=off
  tag scope: W_fan=global
  wires:
  T_fg/1 -> Fan/1(T_fg)
  Sum of Elements/1 -> Fan/2(F_fg)
  Fi_fg/1 -> Out2/1, Sum of Elements/1
  Fan/1(T_out) -> Out1/1
  Fan/2(W_el) -> [W_fan]

== system Furnace/Plant2/Flue-gas stack ==
  T_fg : Inport
  Fi_fg : Inport  Port=2
  F_fg : Scope
  T_fg_fromECO : Scope
  wires:
  T_fg/1 -> T_fg_fromECO/1
  Fi_fg/1 -> F_fg/1

== system Furnace/Plant2/Free board ==
  Fi_in : Inport
  T_in : Inport  Port=2
  Q_rad : Inport  Port=3
  F_flyash_cell : Inport  Port=4
  F_aII_in : Inport  Port=5
  T_aII_in : Inport  Port=6
  DIFF_Free Board : MATLAB Function  TreatAsAtomicUnit=on
  M_fg_part : Integrator  InitialCondition=[k.M_fg_IC.*k.w_a(1:k.nc_gas-1)]
  M_steel : Constant  Value=k.M_steel_FB
  Mw_gas : Constant  Value=k.Mw_gas
  Scope : Scope
  Sum of Elements : Sum  Inputs=+
  T_amb : Constant  Value=k.T_amb
  T_fg : Integrator  InitialCondition=k.T_0
  To Workspace : ToWorkspace  VariableName=Y_H2O  SaveFormat=Structure With Time  SampleTime=-1
  V_FB : Constant  Value=k.V_FreeBoard
  cp_fg : Constant  Value=k.cp_fg
  cp_steel : Constant  Value=k.cp_steel
  p_amb : Constant  Value=k.p_amb
  T_fg_out : Outport  VectorParamsAs1DForOutWhenUnconnected=off
  Fi_fg_to_boiler : Outport  Port=2  VectorParamsAs1DForOutWhenUnconnected=off
  F_flyash_tot : Outport  Port=3  VectorParamsAs1DForOutWhenUnconnected=off
  wires:
  T_in/1 -> DIFF_Free Board/4(T_in)  "T_in"
  p_amb/1 -> DIFF_Free Board/8(p_amb)
  DIFF_Free Board/1(dMfg_dt_int) -> M_fg_part/1
  DIFF_Free Board/2(dTfg_dt) -> T_fg/1
  M_fg_part/1 -> DIFF_Free Board/1(M_fg_int)
  DIFF_Free Board/4(M_fg) -> Scope/1
  Q_rad/1 -> DIFF_Free Board/7(Q_rad)  "Q_rad"
  Fi_in/1 -> DIFF_Free Board/3(Fi_in)
  DIFF_Free Board/5(Y_H2O) -> To Workspace/1
  T_fg/1 -> DIFF_Free Board/2(T_fg), T_fg_out/1
  DIFF_Free Board/3(Fi_fg_out) -> Fi_fg_to_boiler/1
  V_FB/1 -> DIFF_Free Board/9(V_FreeBoard)
  Mw_gas/1 -> DIFF_Free Board/10(Mw_gas)
  T_amb/1 -> DIFF_Free Board/11(T_amb)
  cp_fg/1 -> DIFF_Free Board/12(cp_fg)
  cp_steel/1 -> DIFF_Free Board/13(cp_steel)
  M_steel/1 -> DIFF_Free Board/14(M_steel_FB)
  F_flyash_cell/1 -> Sum of Elements/1
  Sum of Elements/1 -> F_flyash_tot/1
  F_aII_in/1 -> DIFF_Free Board/5(F_aII)
  T_aII_in/1 -> DIFF_Free Board/6(T_aII)

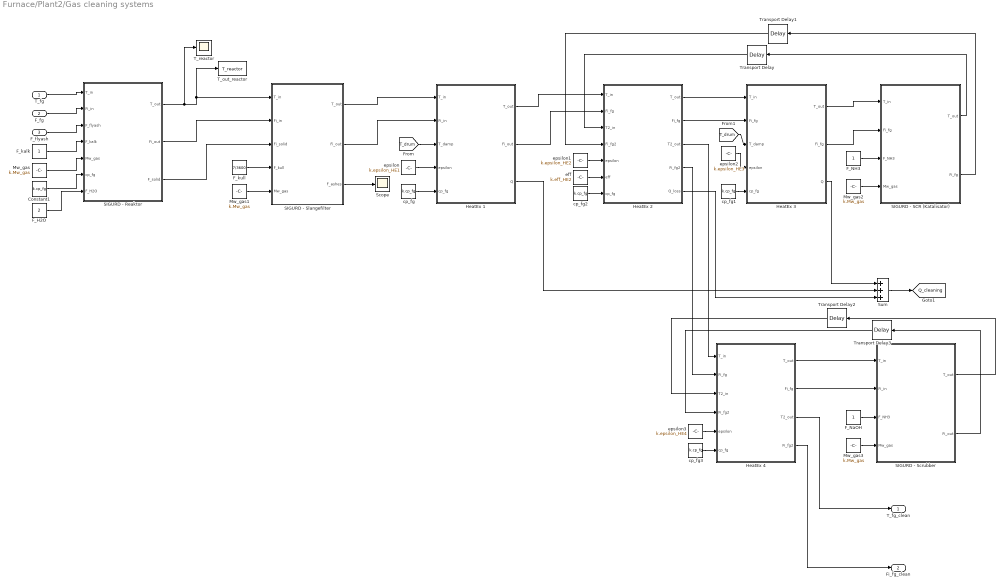
== system Furnace/Plant2/Gas cleaning systems ==
  T_fg : Inport
  F_fg : Inport  Port=2
  F_flyash : Inport  Port=3
  Constant1 : Constant  Value=k.cp_fg
  F_H2O : Constant  Value=2
  F_NH3 : Constant
  F_NaOH : Constant
  F_kalk : Constant
  F_kull : Constant  Value=7/3600
  HeatEx 1 : MATLAB Function  TreatAsAtomicUnit=on
  HeatEx 2 : MATLAB Function  TreatAsAtomicUnit=on
  HeatEx 3 : MATLAB Function  TreatAsAtomicUnit=on
  HeatEx 4 : MATLAB Function  TreatAsAtomicUnit=on
  Mw_gas{,1..3} (4 alike) : Constant  Value=k.Mw_gas
  SIGURD - Reaktor : MATLAB Function  TreatAsAtomicUnit=on
  SIGURD - SCR (Katalisator) : MATLAB Function  TreatAsAtomicUnit=on
  SIGURD - Scrubber : MATLAB Function  TreatAsAtomicUnit=on
  SIGURD - Slangefilter : MATLAB Function  TreatAsAtomicUnit=on
  Scope : Scope
  Sum : Sum  Inputs=+++
  T_out_reactor : ToWorkspace  VariableName=T_reactor  SaveFormat=Timeseries  SampleTime=-1
  T_reactor : Scope
  Transport Delay : TransportDelay  DelayTime=2  InitialOutput=k.T_amb
  Transport Delay1 : TransportDelay  DelayTime=2  InitialOutput=ones(k.nc_gas,1)
  Transport Delay2 : TransportDelay  DelayTime=2  InitialOutput=k.T_amb
  Transport Delay3 : TransportDelay  DelayTime=2  InitialOutput=ones(k.nc_gas,1)
  cp_fg{,1..3} (4 alike) : Constant  Value=k.cp_fg
  eff : Constant  Value=k.eff_HE2
  epsilon : Constant  Value=k.epsilon_HE1
  epsilon1 : Constant  Value=k.epsilon_HE2
  epsilon2 : Constant  Value=k.epsilon_HE3
  epsilon3 : Constant  Value=k.epsilon_HE4
  T_fg_clean : Outport  VectorParamsAs1DForOutWhenUnconnected=off
  Fi_fg_clean : Outport  Port=2  VectorParamsAs1DForOutWhenUnconnected=off
  tag scope: Q_cleaning=global
  wires:
  T_fg/1 -> SIGURD - Reaktor/1(T_in)
  F_fg/1 -> SIGURD - Reaktor/2(Fi_in)
  SIGURD - Reaktor/1(T_out) -> T_reactor/1, T_out_reactor/1, SIGURD - Slangefilter/1(T_in)
  SIGURD - Reaktor/2(Fi_out) -> SIGURD - Slangefilter/2(Fi_in)
  F_kalk/1 -> SIGURD - Reaktor/4(F_kalk)
  Mw_gas/1 -> SIGURD - Reaktor/5(Mw_gas)
  F_kull/1 -> SIGURD - Slangefilter/4(F_kull)
  Mw_gas1/1 -> SIGURD - Slangefilter/5(Mw_gas)
  SIGURD - Slangefilter/1(T_out) -> HeatEx 1/1(T_in)
  SIGURD - Slangefilter/2(Fi_out) -> HeatEx 1/2(Fi_in)
  [T_drum] -> HeatEx 1/3(T_damp)
  epsilon/1 -> HeatEx 1/4(epsilon)
  HeatEx 1/1(T_out) -> HeatEx 2/1(T_in)
  HeatEx 1/2(Fi_out) -> HeatEx 2/2("Fi_fg ")
  HeatEx 2/1(T_out) -> HeatEx 3/1(T_in)
  HeatEx 2/2(Fi_fg) -> HeatEx 3/2("Fi_fg ")
  [T_drum] -> HeatEx 3/3(T_damp)
  epsilon1/1 -> HeatEx 2/5(epsilon)
  epsilon2/1 -> HeatEx 3/4(epsilon)
  HeatEx 1/3(Q) -> Sum/2
  HeatEx 3/3(Q) -> Sum/1
  HeatEx 3/1(T_out) -> SIGURD - SCR (Katalisator)/1(T_in)
  HeatEx 3/2(Fi_fg) -> SIGURD - SCR (Katalisator)/2("Fi_fg ")
  F_NH3/1 -> SIGURD - SCR (Katalisator)/3(F_NH3)
  Mw_gas2/1 -> SIGURD - SCR (Katalisator)/4(Mw_gas)
  SIGURD - SCR (Katalisator)/1(T_out) -> Transport Delay/1
  SIGURD - SCR (Katalisator)/2(Fi_fg) -> Transport Delay1/1
  HeatEx 2/3(T2_out) -> HeatEx 4/1(T_in)
  HeatEx 2/4(Fi_fg2) -> HeatEx 4/2("Fi_fg ")
  epsilon3/1 -> HeatEx 4/5(epsilon)
  HeatEx 4/1(T_out) -> SIGURD - Scrubber/1(T_in)
  HeatEx 4/2(Fi_fg) -> SIGURD - Scrubber/2(Fi_in)
  SIGURD - Scrubber/1(T_out) -> Transport Delay2/1
  SIGURD - Scrubber/2(Fi_out) -> Transport Delay3/1
  F_NaOH/1 -> SIGURD - Scrubber/3(F_NH3)
  Mw_gas3/1 -> SIGURD - Scrubber/4(Mw_gas)
  HeatEx 4/3(T2_out) -> T_fg_clean/1
  HeatEx 4/4(Fi_fg2) -> Fi_fg_clean/1
  SIGURD - Slangefilter/3(F_ashes) -> Scope/1
  cp_fg/1 -> HeatEx 1/5(cp_fg)
  cp_fg1/1 -> HeatEx 3/5(cp_fg)
  cp_fg2/1 -> HeatEx 2/7(cp_fg)
  Constant1/1 -> SIGURD - Reaktor/6(cp_fg)
  SIGURD - Reaktor/3(F_solid) -> SIGURD - Slangefilter/3(Fi_solid)
  F_flyash/1 -> SIGURD - Reaktor/3(F_flyash)
  Transport Delay/1 -> HeatEx 2/3(T2_in)
  Transport Delay1/1 -> HeatEx 2/4("Fi_fg2 ")
  Transport Delay2/1 -> HeatEx 4/3(T2_in)
  Transport Delay3/1 -> HeatEx 4/4("Fi_fg2 ")
  cp_fg3/1 -> HeatEx 4/6(cp_fg)
  eff/1 -> HeatEx 2/6(eff)
  Sum/1 -> [Q_cleaning]
  HeatEx 2/5(Q_loss) -> Sum/3
  F_H2O/1 -> SIGURD - Reaktor/7(F_H2O)

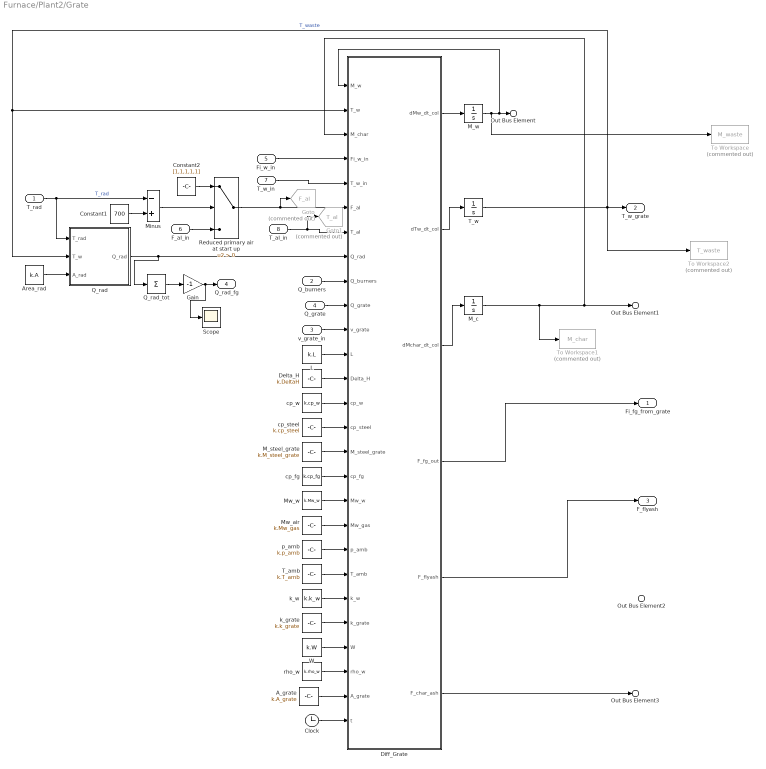
== system Furnace/Plant2/Grate ==
  T_rad : Inport
  Q_burners : Inport  Port=2
  v_grate_in : Inport  Port=3
  Q_grate : Inport  Port=4
  Fi_w_in : Inport  Port=5
  F_aI_in : Inport  Port=6
  T_w_in : Inport  Port=7
  T_aI_in : Inport  Port=8
  A_grate : Constant  Value=k.A_grate
  Area_rad : Constant  Value=k.A
  Clock : Clock
  Constant1 : Constant  Value=700
  Constant2 : Constant  Value=[1,1,1,1,1]
  Delta_H : Constant  Value=k.DeltaH
  Diff_Grate : MATLAB Function  TreatAsAtomicUnit=on
  Gain : Gain  Gain=-1
  Goto : Goto  Commented=on  GotoTag=F_aI  TagVisibility=global
  Goto1 : Goto  Commented=on  GotoTag=T_aI  TagVisibility=global
  L : Constant  Value=k.L
  M_c : Integrator  InitialCondition=zeros(k.n_cell,1)
  M_steel_grate : Constant  Value=k.M_steel_grate
  M_w : Integrator  InitialCondition=zeros(k.n_cell.*(k.nc_w+2),1)
  Minus : Sum  Inputs=-+
  Mw_air : Constant  Value=k.Mw_gas
  Mw_w : Constant  Value=k.Mw_w
  Q_rad : Subsystem
  Q_rad_tot : Sum  Inputs=+
  Reduced primary air at start up : Switch  Criteria=u2 > Threshold
  Scope : Scope
  T_amb : Constant  Value=k.T_amb
  T_w : Integrator  InitialCondition=k.T_amb.*ones(k.n_cell,1)
  To Workspace : ToWorkspace  Commented=on  VariableName=M_waste  SaveFormat=Structure With Time  SampleTime=-1
  To Workspace1 : ToWorkspace  Commented=on  VariableName=M_char  SaveFormat=Structure With Time  SampleTime=-1
  To Workspace2 : ToWorkspace  Commented=on  VariableName=T_waste  SaveFormat=Structure With Time  SampleTime=-1
  W : Constant  Value=k.W
  cp_fg : Constant  Value=k.cp_fg
  cp_steel : Constant  Value=k.cp_steel
  cp_w : Constant  Value=k.cp_w
  k_grate : Constant  Value=k.k_grate
  k_w : Constant  Value=k.k_w
  p_amb : Constant  Value=k.p_amb
  rho_w : Constant  Value=k.rho_w
  Fi_fg_from_grate : Outport  VectorParamsAs1DForOutWhenUnconnected=off
  T_w_grate : Outport  Port=2  VectorParamsAs1DForOutWhenUnconnected=off
  F_flyash : Outport  Port=3  VectorParamsAs1DForOutWhenUnconnected=off
  Q_rad_fg : Outport  Port=4  VectorParamsAs1DForOutWhenUnconnected=off
  Out Bus Element : Outport  Port=5  VectorParamsAs1DForOutWhenUnconnected=off  PortName=OutBus  Element=M_w_grate
  Out Bus Element1 : Outport  Port=5  VectorParamsAs1DForOutWhenUnconnected=off  PortName=OutBus  Element=M_char
  Out Bus Element2 : Outport  Port=5  VectorParamsAs1DForOutWhenUnconnected=off  PortName=OutBus  Element=F_w_ash
  Out Bus Element3 : Outport  Port=5  VectorParamsAs1DForOutWhenUnconnected=off  PortName=OutBus  Element=F_char_ash
  wires:
  Diff_Grate/2(dTw_dt_col) -> T_w/1
  Area_rad/1 -> Q_rad/3(A_rad)
  M_w/1 -> To Workspace/1, Out Bus Element/1, Diff_Grate/1(M_w)
  T_aI_in/1 -> Goto1/1, Diff_Grate/7(T_aI)
  Q_rad/1(Q_rad) -> Q_rad_tot/1, Diff_Grate/8(Q_rad)
  Diff_Grate/1(dMw_dt_col) -> M_w/1
  T_w/1 -> Diff_Grate/2(T_w), Q_rad/2(T_w), T_w_grate/1, To Workspace2/1  "T_waste"
  ? -> Out Bus Element2/1
  Diff_Grate/4(F_fg_out) -> Fi_fg_from_grate/1
  Diff_Grate/3(dMchar_dt_col) -> M_c/1
  M_c/1 -> To Workspace1/1, Out Bus Element1/1, Diff_Grate/3(M_char)
  Diff_Grate/6(F_char_ash) -> Out Bus Element3/1
  Q_rad_tot/1 -> Gain/1
  Gain/1 -> Scope/1, Q_rad_fg/1
  Q_burners/1 -> Diff_Grate/9(Q_burners)
  Clock/1 -> Diff_Grate/27(t)
  Q_grate/1 -> Diff_Grate/10(Q_grate)
  T_rad/1 -> Minus/1, Q_rad/1(T_rad)  "T_rad"
  Constant1/1 -> Minus/2
  Minus/1 -> Reduced primary air at start up/2
  F_aI_in/1 -> Reduced primary air at start up/3
  Reduced primary air at start up/1 -> Goto/1, Diff_Grate/6(F_aI)
  Constant2/1 -> Reduced primary air at start up/1
  L/1 -> Diff_Grate/12(L)
  Delta_H/1 -> Diff_Grate/13(Delta_H)
  cp_w/1 -> Diff_Grate/14(cp_w)
  cp_steel/1 -> Diff_Grate/15(cp_steel)
  M_steel_grate/1 -> Diff_Grate/16(M_steel_grate)
  cp_fg/1 -> Diff_Grate/17(cp_fg)
  Mw_w/1 -> Diff_Grate/18(Mw_w)
  Mw_air/1 -> Diff_Grate/19(Mw_gas)
  p_amb/1 -> Diff_Grate/20(p_amb)
  T_amb/1 -> Diff_Grate/21(T_amb)
  k_w/1 -> Diff_Grate/22(k_w)
  k_grate/1 -> Diff_Grate/23(k_grate)
  W/1 -> Diff_Grate/24(W)
  rho_w/1 -> Diff_Grate/25(rho_w)
  A_grate/1 -> Diff_Grate/26(A_grate)
  Diff_Grate/5(F_flyash) -> F_flyash/1
  v_grate_in/1 -> Diff_Grate/11(v_grate)
  Fi_w_in/1 -> Diff_Grate/4(Fi_w_in)
  T_w_in/1 -> Diff_Grate/5(T_w_in)

== system Furnace/Plant2/Hot water to district heating ==
  In1 : Inport
  T_district : Scope
  wires:
  In1/1 -> T_district/1
